simulink model "plant2"  (R2016b)
settings: Solver=VariableStepAuto  StartTime=0.0  StopTime=10.0  RelTol=1e-3
undefined symbols (not defined in the file): Earth, initialValues, LD, WGS84
libraries: aerolibbdyn x2, aerolib6dof2 x1, aerolibtransform2 x1, aerolibasang x1
settings Model: Creator=Uxío  LastModifiedBy=Uxío

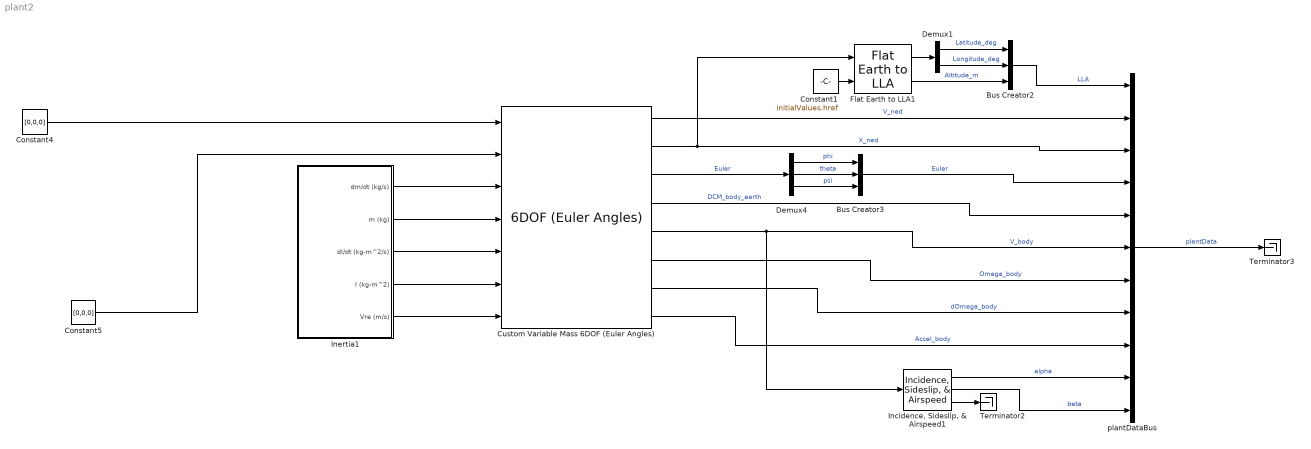
== system plant2 ==
  Bus Creator2 : BusCreator  Inputs=3
  Bus Creator3 : BusCreator  Inputs=3
  Constant1 : Constant  Value=initialValues.href
  Constant4 : Constant  Value=[0,0,0]
  Constant5 : Constant  Value=[0,0,0]
  Custom Variable Mass 6DOF (Euler Angles) : aerolib6dof2/6DOF (Euler Angles)  units=Metric (MKS)  mtype=Custom Variable  rep=Euler Angles  xme_0=[initialValues.Xe0 initialValues.Ye0 initialValues.Ze0]  Vm_0=[initialValues.u0 initialValues.v0 initialValues.w0]  eul_0=[initialValues.roll0 initialValues.pitch0 initialValues.yaw0]  pm_0=[initialValues.p0 initialValues.q0 initialValues.r0]  mass_0=1.0  mass_e=0.5  mass_f=2.0  inertia=eye(3)  inertia_e=eye(3)  inertia_f=2*eye(3)  k_quat=1.0  vre_flag=on
  Demux1 : Demux  Outputs=2
  Demux4 : Demux  Outputs=3
  Flat Earth to LLA1 : aerolibtransform2/Flat Earth to LLA  units=Metric (MKS)  ptype=Earth (WGS84)  F=1/298.257223563  R=6378137  LL0=initialValues.LatLong0  psi=initialValues.heading0
  "Incidence, Sideslip, & Airspeed1" : aerolibasang/Incidence, Sideslip, & Airspeed
  Inertia1 : Subsystem
  Terminator2 : Terminator
  Terminator3 : Terminator
  plantDataBus : BusCreator  Inputs=11
  wires:
  Inertia1/1(dm/dt (kg/s)) -> Custom Variable Mass 6DOF (Euler Angles)/3
  Inertia1/2(m (kg)) -> Custom Variable Mass 6DOF (Euler Angles)/4
  Inertia1/3(dI/dt (kg-m^2/s)) -> Custom Variable Mass 6DOF (Euler Angles)/5
  Inertia1/4(I (kg-m^2)) -> Custom Variable Mass 6DOF (Euler Angles)/6
  Inertia1/5(Vre (m/s)) -> Custom Variable Mass 6DOF (Euler Angles)/7
  Constant1/1 -> Flat Earth to LLA1/2
  Flat Earth to LLA1/2 -> Bus Creator2/3  "Altitude_m"
  Flat Earth to LLA1/1 -> Demux1/1
  Demux1/1 -> Bus Creator2/1  "Latitude_deg"
  Demux1/2 -> Bus Creator2/2  "Longitude_deg"
  Custom Variable Mass 6DOF (Euler Angles)/1 -> plantDataBus/2  "V_ned"
  Custom Variable Mass 6DOF (Euler Angles)/2 -> plantDataBus/3, Flat Earth to LLA1/1  "X_ned"
  Custom Variable Mass 6DOF (Euler Angles)/4 -> plantDataBus/5  "DCM_body_earth"
  Custom Variable Mass 6DOF (Euler Angles)/5 -> "Incidence, Sideslip, & Airspeed1"/1, plantDataBus/6  "V_body"
  Custom Variable Mass 6DOF (Euler Angles)/6 -> plantDataBus/7  "Omega_body"
  Custom Variable Mass 6DOF (Euler Angles)/7 -> plantDataBus/8  "dOmega_body"
  Bus Creator2/1 -> plantDataBus/1  "LLA"
  plantDataBus/1 -> Terminator3/1  "plantData"
  Custom Variable Mass 6DOF (Euler Angles)/8 -> plantDataBus/9  "Accel_body"
  "Incidence, Sideslip, & Airspeed1"/1 -> plantDataBus/10  "alpha"
  "Incidence, Sideslip, & Airspeed1"/2 -> plantDataBus/11  "beta"
  "Incidence, Sideslip, & Airspeed1"/3 -> Terminator2/1
  Custom Variable Mass 6DOF (Euler Angles)/3 -> Demux4/1  "Euler"
  Demux4/1 -> Bus Creator3/1  "phi"
  Demux4/2 -> Bus Creator3/2  "theta"
  Demux4/3 -> Bus Creator3/3  "psi"
  Bus Creator3/1 -> plantDataBus/4  "Euler"
  Constant4/1 -> Custom Variable Mass 6DOF (Euler Angles)/1
  Constant5/1 -> Custom Variable Mass 6DOF (Euler Angles)/2

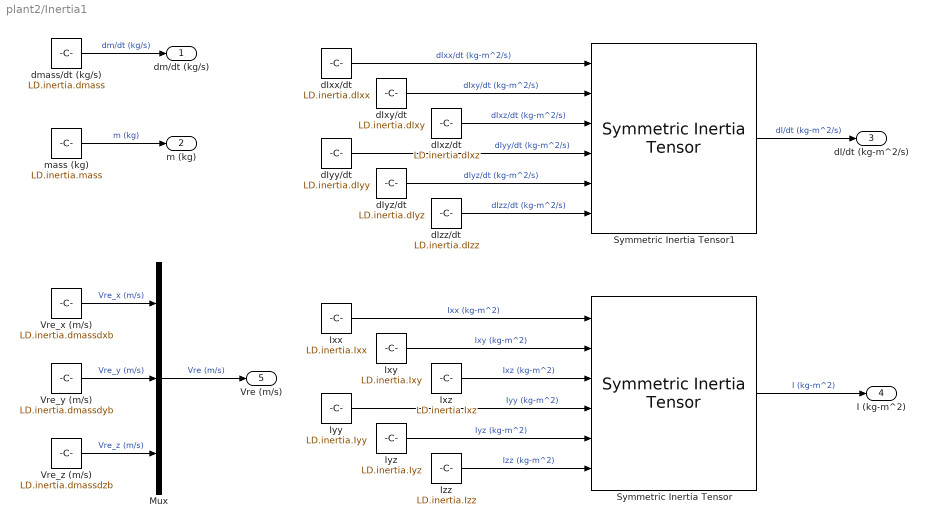
== system plant2/Inertia1 ==
  Ixx : Constant  Value=LD.inertia.Ixx
  Ixy : Constant  Value=LD.inertia.Ixy
  Ixz : Constant  Value=LD.inertia.Ixz
  Iyy : Constant  Value=LD.inertia.Iyy
  Iyz : Constant  Value=LD.inertia.Iyz
  Izz : Constant  Value=LD.inertia.Izz
  Mux : Mux  Inputs=3
  Symmetric Inertia Tensor : aerolibbdyn/Symmetric Inertia Tensor
  Symmetric Inertia Tensor1 : aerolibbdyn/Symmetric Inertia Tensor
  Vre_x (m/s) : Constant  Value=LD.inertia.dmassdxb
  Vre_y (m/s) : Constant  Value=LD.inertia.dmassdyb
  Vre_z (m/s) : Constant  Value=LD.inertia.dmassdzb
  dIxx/dt : Constant  Value=LD.inertia.dIxx
  dIxy/dt : Constant  Value=LD.inertia.dIxy
  dIxz/dt : Constant  Value=LD.inertia.dIxz
  dIyy/dt : Constant  Value=LD.inertia.dIyy
  dIyz/dt : Constant  Value=LD.inertia.dIyz
  dIzz/dt : Constant  Value=LD.inertia.dIzz
  dmass/dt (kg/s) : Constant  Value=LD.inertia.dmass
  mass (kg) : Constant  Value=LD.inertia.mass
  dm/dt (kg/s) : Outport  Unit=kg/s
  m (kg) : Outport  Port=2  Unit=kg
  dI/dt (kg-m^2/s) : Outport  Port=3  Unit=kg*meter^2/s
  I (kg-m^2) : Outport  Port=4  Unit=kg*meter*meter
  Vre (m/s) : Outport  Port=5  Unit=meter/s
  wires:
  Symmetric Inertia Tensor/1 -> I (kg-m^2)/1  "I (kg-m^2)"
  Symmetric Inertia Tensor1/1 -> dI/dt (kg-m^2/s)/1  "dI/dt (kg-m^2/s)"
  dIxx/dt/1 -> Symmetric Inertia Tensor1/1  "dIxx/dt (kg-m^2/s)"
  dIxz/dt/1 -> Symmetric Inertia Tensor1/3  "dIxz/dt (kg-m^2/s)"
  dIxy/dt/1 -> Symmetric Inertia Tensor1/2  "dIxy/dt (kg-m^2/s)"
  dIyy/dt/1 -> Symmetric Inertia Tensor1/4  "dIyy/dt (kg-m^2/s)"
  dIzz/dt/1 -> Symmetric Inertia Tensor1/6  "dIzz/dt (kg-m^2/s)"
  dIyz/dt/1 -> Symmetric Inertia Tensor1/5  "dIyz/dt (kg-m^2/s)"
  Ixx/1 -> Symmetric Inertia Tensor/1  "Ixx (kg-m^2)"
  Ixz/1 -> Symmetric Inertia Tensor/3  "Ixz (kg-m^2)"
  Ixy/1 -> Symmetric Inertia Tensor/2  "Ixy (kg-m^2)"
  Iyy/1 -> Symmetric Inertia Tensor/4  "Iyy (kg-m^2)"
  Izz/1 -> Symmetric Inertia Tensor/6  "Izz (kg-m^2)"
  Iyz/1 -> Symmetric Inertia Tensor/5  "Iyz (kg-m^2)"
  mass (kg)/1 -> m (kg)/1  "m (kg)"
  dmass/dt (kg/s)/1 -> dm/dt (kg/s)/1  "dm/dt (kg/s)"
  Vre_x (m/s)/1 -> Mux/1  "Vre_x (m/s)"
  Vre_z (m/s)/1 -> Mux/3  "Vre_z (m/s)"
  Vre_y (m/s)/1 -> Mux/2  "Vre_y (m/s)"
  Mux/1 -> Vre (m/s)/1  "Vre (m/s)"
